simulink model "Voltage_Vector_with_script_fianl"  (R2024b)
settings: Solver=FixedStepAuto  StartTime=0.0  StopTime=0.5  FixedStep=1e-5  RelTol=1e-3
model workspace (MAT data in the model file):
  Cap = 0.004
  FL = 0.025
  Indcut = 0.005
  Initial_Voltage = 125
  R_Load = 1000
  V_dc = 300
  Vd = 125
  Vl = 400
  c = 125
  cap = 7.07e-05
  f_o = 50
  f_s = 5000
libraries: spsIGBTDiodeLib x72, spsSeriesRLCBranchLib x48, spsMultimeterLib x9, spsRMSLib x7, spsThreePhaseBreakerLib x6, spsTHDLib x6, spsThreePhaseSeriesRLCLoadLib x4, spsGroundLib x3, spsCurrentMeasurementLib x2, spsDCVoltageSourceLib x2, spsThreePhaseVIMeasurementLib x2, slpidlib x1
(part 3 of 3)

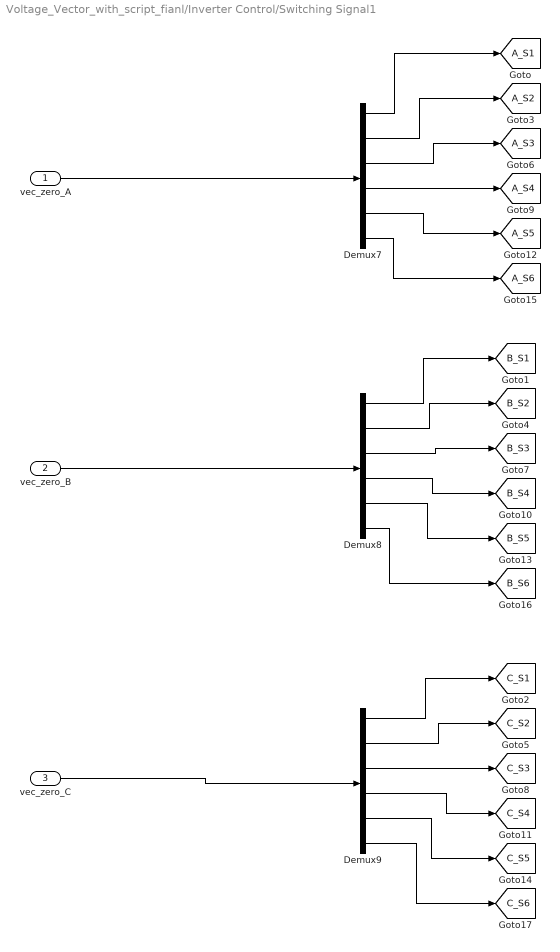
== system Voltage_Vector_with_script_fianl/Inverter Control/Switching Signal1 ==
  vec_zero_A : Inport
  vec_zero_B : Inport  Port=2
  vec_zero_C : Inport  Port=3
  Demux7 : Demux  Outputs=6
  Demux8 : Demux  Outputs=6
  Demux9 : Demux  Outputs=6
  tag scope: A_S1=global, A_S2=global, A_S3=global, A_S4=global, A_S5=global, A_S6=global, B_S1=global, B_S2=global, B_S3=global, B_S4=global, B_S5=global, B_S6=global, C_S1=global, C_S2=global, C_S3=global, C_S4=global, C_S5=global, C_S6=global
  wires:
  vec_zero_B/1 -> Demux8/1
  vec_zero_A/1 -> Demux7/1
  Demux8/2 -> [B_S2]
  Demux9/3 -> [C_S3]
  Demux8/4 -> [B_S4]
  vec_zero_C/1 -> Demux9/1
  Demux9/6 -> [C_S6]
  Demux7/2 -> [A_S2]
  Demux9/4 -> [C_S4]
  Demux7/4 -> [A_S4]
  Demux9/5 -> [C_S5]
  Demux9/1 -> [C_S1]
  Demux8/5 -> [B_S5]
  Demux7/3 -> [A_S3]
  Demux7/6 -> [A_S6]
  Demux9/2 -> [C_S2]
  Demux8/1 -> [B_S1]
  Demux8/3 -> [B_S3]
  Demux7/1 -> [A_S1]
  Demux8/6 -> [B_S6]
  Demux7/5 -> [A_S5]

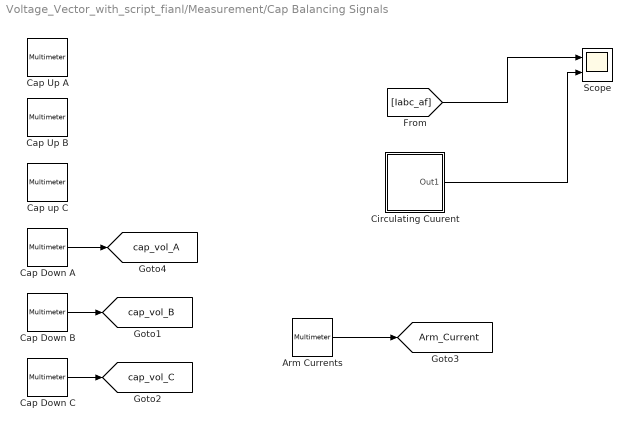
== system Voltage_Vector_with_script_fianl/Measurement/Cap Balancing Signals ==
  Arm Currents : spsMultimeterLib/Multimeter  L=86  sel=[46 48 50]  yselected={}  Gain=[1 1 1]  OutputType=Complex  PlotAtSimulationStop=on  PhasorSimulation=off
  Cap Down A : spsMultimeterLib/Multimeter  L=86  sel=[34 37 40 10 13 16]  yselected={}  Gain=[1 1 1 1 1 1]  OutputType=Complex  PlotAtSimulationStop=on  PhasorSimulation=off
  Cap Down B : spsMultimeterLib/Multimeter  L=86  sel=[35 38 41 11 14 17]  yselected={}  Gain=[1 1 1 1 1 1]  OutputType=Complex  PlotAtSimulationStop=on  PhasorSimulation=off
  Cap Down C : spsMultimeterLib/Multimeter  L=86  sel=[36 39 42 12 15 18]  yselected={}  Gain=[1 1 1 1 1 1]  OutputType=Complex  PlotAtSimulationStop=on  PhasorSimulation=off
  Cap Up A : spsMultimeterLib/Multimeter  L=86  sel=[7 19 22 25 28 31]  yselected={}  Gain=[1 1 1 1 1 1]  OutputType=Complex  PlotAtSimulationStop=off  PhasorSimulation=off
  Cap Up B : spsMultimeterLib/Multimeter  L=86  sel=[8 20 23 26 29 32]  yselected={}  Gain=[1 1 1 1 1 1]  OutputType=Complex  PlotAtSimulationStop=off  PhasorSimulation=off
  Cap up C : spsMultimeterLib/Multimeter  L=86  sel=[9 21 24 27 30 33]  yselected={}  Gain=[1 1 1 1 1 1]  OutputType=Complex  PlotAtSimulationStop=off  PhasorSimulation=off
  Circulating Cuurent : Subsystem
  Scope : Scope  NumInputPorts=2
  tag scope: Arm_Current=global, cap_vol_A=global, cap_vol_B=global, cap_vol_C=global
  wires:
  Cap Down A/1 -> [cap_vol_A]
  Cap Down B/1 -> [cap_vol_B]
  Cap Down C/1 -> [cap_vol_C]
  Arm Currents/1 -> [Arm_Current]
  [Iabc_af] -> Scope/1
  Circulating Cuurent/1(Out1) -> Scope/2

== system Voltage_Vector_with_script_fianl/Measurement/Current Measurements ==
  After Filtering : Subsystem
  Before Filtering : Subsystem

== system Voltage_Vector_with_script_fianl/Measurement/Voltage Measurements ==
  After Filtering : Subsystem
  Before Filtering : Subsystem
  Subsystem : Subsystem

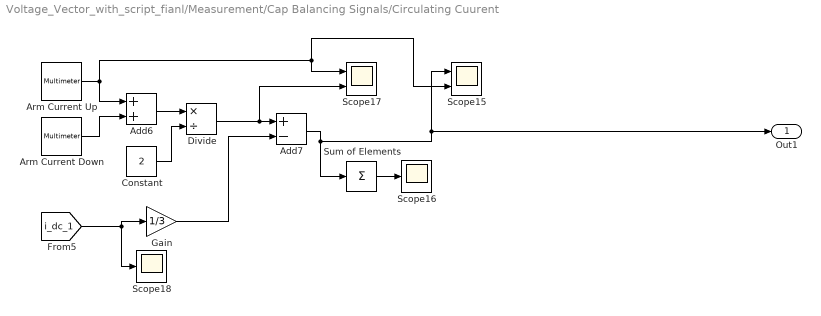
== system Voltage_Vector_with_script_fianl/Measurement/Cap Balancing Signals/Circulating Cuurent ==
  Add6 : Sum
  Add7 : Sum  Inputs=+-
  Arm Current Down : spsMultimeterLib/Multimeter  L=86  sel=[46 48 50]  yselected={}  Gain=[1 1 1]  OutputType=Complex  PlotAtSimulationStop=on  PhasorSimulation=off
  Arm Current Up : spsMultimeterLib/Multimeter  L=86  sel=[45 47 49]  yselected={}  Gain=[1 1 1]  OutputType=Complex  PlotAtSimulationStop=off  PhasorSimulation=off
  Constant : Constant  Value=2
  Divide : Product  Inputs=*/
  Gain : Gain  Gain=1/3
  Scope15 : Scope  NumInputPorts=2
  Scope16 : Scope
  Scope17 : Scope  NumInputPorts=2
  Scope18 : Scope
  Sum of Elements : Sum  Inputs=+
  Out1 : Outport
  wires:
  Gain/1 -> Add7/2
  Divide/1 -> Scope17/2, Add7/1
  Arm Current Up/1 -> Scope17/1, Scope15/2, Add6/1
  Add7/1 -> Sum of Elements/1, Out1/1, Scope15/1
  [i_dc_1] -> Gain/1, Scope18/1
  Add6/1 -> Divide/1
  Sum of Elements/1 -> Scope16/1
  Arm Current Down/1 -> Add6/2
  Constant/1 -> Divide/2

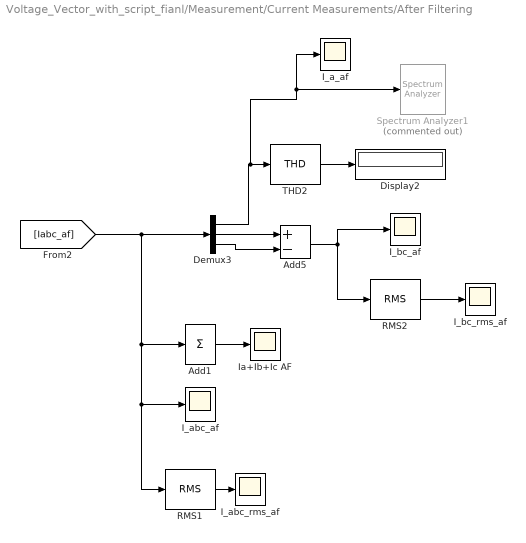
== system Voltage_Vector_with_script_fianl/Measurement/Current Measurements/After Filtering ==
  Add1 : Sum  Inputs=+
  Add5 : Sum  Inputs=+-
  Demux3 : Demux  Outputs=3
  Display2 : Display
  I_a_af : Scope
  I_abc_af : Scope
  I_abc_rms_af : Scope
  I_bc_af : Scope
  I_bc_rms_af : Scope
  Ia+Ib+Ic AF : Scope
  RMS1 : spsRMSLib/RMS  TrueRMS=on  Freq=50  RMSInit=120  Ts=0
  RMS2 : spsRMSLib/RMS  TrueRMS=on  Freq=50  RMSInit=120  Ts=0
  Spectrum Analyzer1 : SpectrumAnalyzer  Commented=on  WindowPosition=[1.000000,1.000000,1536.000000,840.000000,]  ScopeFrameLocation=window  ViewType=Spectrum and spectrogram  SampleRateSource=Property  SampleRate=44.1e3  PlotAsTwoSidedSpectrum=off  FrequencyScale=Log  RBW=50  FrequencySpan=Start and stop frequencies  StartFrequency=50  StopFrequency=20e3  YLimits=[-21.67839413,61.32124814]  ColorLimits=[-21.67839413,61.32124814]  SelectedToolstripTab=spectrumAnalyzerToolstrip.measurementsTab
  THD2 : spsTHDLib/THD  Freq=60  Ts=0
  wires:
  RMS1/1 -> I_abc_rms_af/1
  RMS2/1 -> I_bc_rms_af/1
  Demux3/2 -> Add5/1
  Add1/1 -> Ia+Ib+Ic AF/1
  Demux3/3 -> Add5/2
  THD2/1 -> Display2/1
  Demux3/1 -> THD2/1, Spectrum Analyzer1/1, I_a_af/1
  [Iabc_af] -> Demux3/1, Add1/1, I_abc_af/1, RMS1/1
  Add5/1 -> I_bc_af/1, RMS2/1

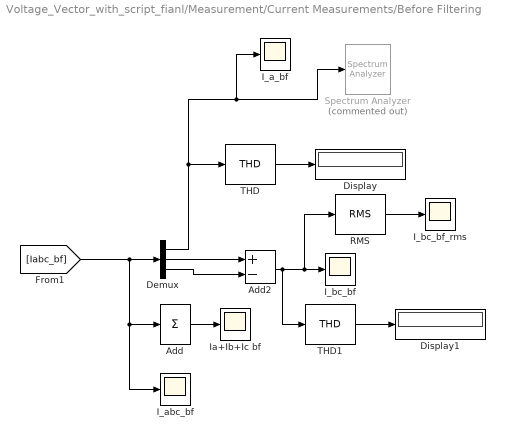
== system Voltage_Vector_with_script_fianl/Measurement/Current Measurements/Before Filtering ==
  Add : Sum  Inputs=+
  Add2 : Sum  Inputs=+-
  Demux : Demux  Outputs=3
  Display : Display
  Display1 : Display
  I_a_bf : Scope
  I_abc_bf : Scope
  I_bc_bf : Scope
  I_bc_bf_rms : Scope
  Ia+Ib+Ic bf : Scope
  RMS : spsRMSLib/RMS  TrueRMS=on  Freq=50  RMSInit=120  Ts=0
  Spectrum Analyzer : SpectrumAnalyzer  Commented=on  WindowPosition=[1.000000,1.000000,1536.000000,840.000000,]  ScopeFrameLocation=window  ViewType=Spectrum and spectrogram  SampleRateSource=Property  SampleRate=44.1e3  PlotAsTwoSidedSpectrum=off  FrequencyScale=Log  RBW=50  FrequencySpan=Start and stop frequencies  StartFrequency=50  StopFrequency=20e3  YLimits=[-37.25091553,62.23523651]  ColorLimits=[-37.25091553,62.23523651]  SelectedToolstripTab=spectrumAnalyzerToolstrip.measurementsTab
  THD : spsTHDLib/THD  Freq=60  Ts=0
  THD1 : spsTHDLib/THD  Freq=60  Ts=0
  wires:
  Add2/1 -> I_bc_bf/1, RMS/1, THD1/1
  THD1/1 -> Display1/1
  Demux/3 -> Add2/2
  Demux/2 -> Add2/1
  RMS/1 -> I_bc_bf_rms/1
  [Iabc_bf] -> Demux/1, Add/1, I_abc_bf/1
  Add/1 -> Ia+Ib+Ic bf/1
  Demux/1 -> THD/1, I_a_bf/1, Spectrum Analyzer/1
  THD/1 -> Display/1

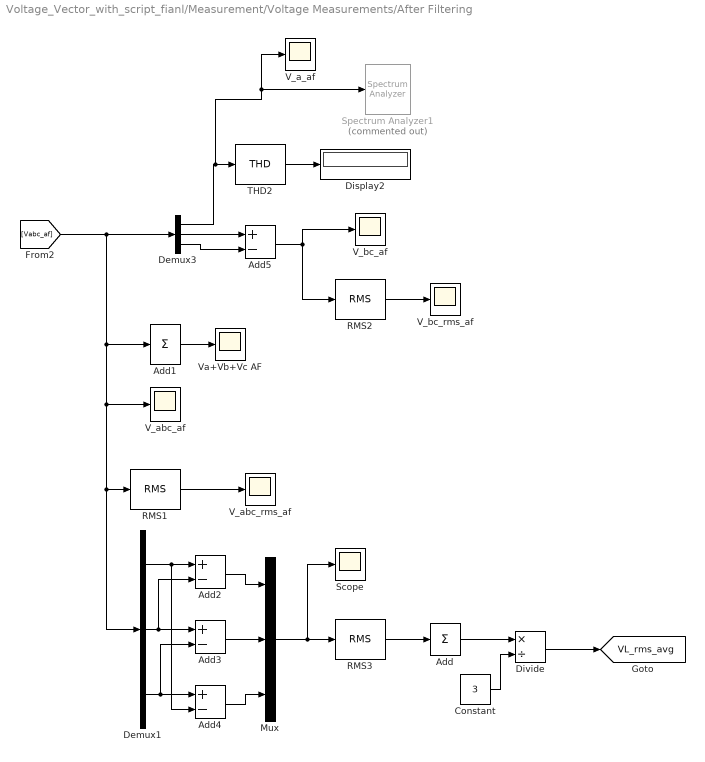
== system Voltage_Vector_with_script_fianl/Measurement/Voltage Measurements/After Filtering ==
  Add : Sum  Inputs=+
  Add1 : Sum  Inputs=+
  Add{2..5} (4 alike) : Sum  Inputs=+-
  Constant : Constant  Value=3
  Demux1 : Demux  Outputs=3
  Demux3 : Demux  Outputs=3
  Display2 : Display
  Divide : Product  Inputs=*/
  Mux : Mux  Inputs=3
  RMS1 : spsRMSLib/RMS  TrueRMS=on  Freq=50  RMSInit=120  Ts=0
  RMS2 : spsRMSLib/RMS  TrueRMS=on  Freq=50  RMSInit=120  Ts=0
  RMS3 : spsRMSLib/RMS  TrueRMS=on  Freq=50  RMSInit=0  Ts=0
  Scope : Scope
  Spectrum Analyzer1 : SpectrumAnalyzer  Commented=on  WindowPosition=[1.000000,1.000000,1536.000000,840.000000,]  ScopeFrameLocation=window  ViewType=Spectrum and spectrogram  SampleRateSource=Property  SampleRate=44.1e3  PlotAsTwoSidedSpectrum=off  FrequencyScale=Log  RBW=50  FrequencySpan=Start and stop frequencies  StartFrequency=50  StopFrequency=20e3  YLimits=[5.0325,80.7583]  ColorLimits=[5.0325,80.7583]  SelectedToolstripTab=spectrumAnalyzerToolstrip.measurementsTab
  THD2 : spsTHDLib/THD  Freq=50  Ts=0
  V_a_af : Scope
  V_abc_af : Scope
  V_abc_rms_af : Scope
  V_bc_af : Scope
  V_bc_rms_af : Scope
  Va+Vb+Vc AF : Scope
  tag scope: VL_rms_avg=global
  wires:
  Add5/1 -> RMS2/1, V_bc_af/1
  [Vabc_af] -> Demux1/1, RMS1/1, V_abc_af/1, Add1/1, Demux3/1
  Demux3/1 -> V_a_af/1, Spectrum Analyzer1/1, THD2/1
  THD2/1 -> Display2/1
  Demux3/3 -> Add5/2
  Add1/1 -> Va+Vb+Vc AF/1
  Demux3/2 -> Add5/1
  RMS2/1 -> V_bc_rms_af/1
  RMS1/1 -> V_abc_rms_af/1
  Add/1 -> Divide/1
  Constant/1 -> Divide/2
  Divide/1 -> [VL_rms_avg]
  Demux1/1 -> Add4/2, Add2/1
  Demux1/2 -> Add2/2, Add3/1
  Demux1/3 -> Add3/2, Add4/1
  Add3/1 -> Mux/2
  Add2/1 -> Mux/1
  Add4/1 -> Mux/3
  Mux/1 -> Scope/1, RMS3/1
  RMS3/1 -> Add/1

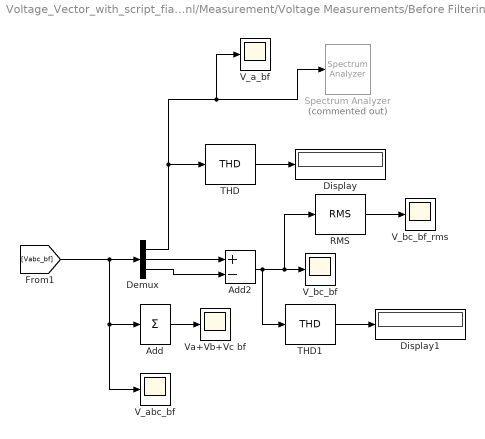
== system Voltage_Vector_with_script_fianl/Measurement/Voltage Measurements/Before Filtering ==
  Add : Sum  Inputs=+
  Add2 : Sum  Inputs=+-
  Demux : Demux  Outputs=3
  Display : Display
  Display1 : Display
  RMS : spsRMSLib/RMS  TrueRMS=on  Freq=50  RMSInit=120  Ts=0
  Spectrum Analyzer : SpectrumAnalyzer  Commented=on  WindowPosition=[1.000000,1.000000,1536.000000,840.000000,]  ScopeFrameLocation=window  ViewType=Spectrum and spectrogram  SampleRateSource=Property  SampleRate=44.1e3  PlotAsTwoSidedSpectrum=off  FrequencyScale=Log  RBW=50  FrequencySpan=Start and stop frequencies  StartFrequency=50  StopFrequency=20e3  YLimits=[-20.56239862,87.43260692]  ColorLimits=[-20.56239862,87.43260692]  SelectedToolstripTab=spectrumAnalyzerToolstrip.measurementsTab
  THD : spsTHDLib/THD  Freq=50  Ts=0
  THD1 : spsTHDLib/THD  Freq=50  Ts=0
  V_a_bf : Scope
  V_abc_bf : Scope
  V_bc_bf : Scope
  V_bc_bf_rms : Scope
  Va+Vb+Vc bf : Scope
  wires:
  THD/1 -> Display/1
  Demux/1 -> Spectrum Analyzer/1, V_a_bf/1, THD/1
  Add/1 -> Va+Vb+Vc bf/1
  [Vabc_bf] -> V_abc_bf/1, Add/1, Demux/1
  RMS/1 -> V_bc_bf_rms/1
  Demux/2 -> Add2/1
  Demux/3 -> Add2/2
  THD1/1 -> Display1/1
  Add2/1 -> THD1/1, RMS/1, V_bc_bf/1

== system Voltage_Vector_with_script_fianl/Measurement/Voltage Measurements/Subsystem ==
  Add : Sum  Inputs=+-
  Add1 : Sum  Inputs=+-
  Demux : Demux  Outputs=3
  Demux1 : Demux  Outputs=3
  Scope : Scope  NumInputPorts=3
  Scope1 : Scope  NumInputPorts=3
  wires:
  [Vabc_af] -> Scope1/1, Demux1/1
  [Vabc_bf] -> Demux/1, Scope/1
  Demux/1 -> Scope/2
  Demux1/1 -> Scope1/2
  Add/1 -> Scope/3
  Add1/1 -> Scope1/3
  Demux/2 -> Add/1
  Demux/3 -> Add/2
  Demux1/2 -> Add1/1
  Demux1/3 -> Add1/2

== matlab function Voltage_Vector_with_script_fianl/Inverter Control/MATLAB Function3 ==
  data: tita_k output; tita input; CV_1 output; CV_2 output; CV_3 output; T output; V_L input; Vd_ input; f input; fs input
function [tita_k, CV_1, CV_2, CV_3, T] = fnc(tita,V_L,Vd_,f,fs)

Ts = 1/fs;

% Transform matrix
A = [1 0 0.5; cos(2*pi/3) sin(2*pi/3) 0.5; cos(4*pi/3) sin(4*pi/3) 0.5]; % Transform matrix
B = [cos(0) cos(2*pi/3) cos(4*pi/3); sin(0) sin(2*pi/3) sin(4*pi/3)];

% Model Parameter
% corner_vec = zeros(1,10);
% dwell_time = zeros(1,4);

% Calculations

r_k = sqrt(6)*V_L / 2;

% tita_k = floor(tita*fs/(f*360))*360*f/fs;
tita_k = tita - mod(tita, 360*f/fs);

x = [r_k*cos(deg2rad(tita_k)); r_k*sin(deg2rad(tita_k)); 0];
V_pole = (2/3)*A*x;
Vnor = V_pole' / Vd_;
% corner_vec(1,1) = tita_k;
% dwell_time(1,1) = tita_k;

% conor vector calculation

CV = Vnor +3;
CV_1 = floor(CV);
error = CV - floor(CV);
[~,i_1] = max(error); % ~ represent the magnitude but ~ neglecte it; i is the index(position), In for loop we can find the magnitude and index
CV_2 = CV_1;
CV_2(i_1) = CV_2(i_1) + 1;
error(i_1) = 0;

[~,i_2] = max(error); % i think max function is not nessaccery , we can you only error
CV_3 = CV_2;
CV_3(i_2) = CV_3(i_2) + 1;
CV_M = [CV_1' CV_2' CV_3'];

temp = [Vd_*B*CV_M; 1 1 1];% first find the Vd*B*CV_M matrix and then add the 1 1 1 row to it.
Y = Ts*[r_k*cos(deg2rad(tita_k));r_k*sin(deg2rad(tita_k)); 1];
T = abs(temp\Y);
           
% corner_vec(1,2:end) = reshape(CV_M, 1, []);
% dwell_time(1,2:end) = T;

== matlab function Voltage_Vector_with_script_fianl/Inverter Control/MATLAB Function2 ==
  data: t input; tita output; fo input; ini_tita input
function tita = fcn(t, fo, ini_tita)

angle = t * fo * 360 + ini_tita;
tita = mod(angle,360);

== matlab function Voltage_Vector_with_script_fianl/Inverter Control/MATLAB Function ==
  data: CV input; vec_zero_A output; cap_vol_a input; cap_vol_b input; cap_vol_c input; arm_cu input; vec_zero_B output; vec_zero_C output
function [vec_zero_A,vec_zero_B,vec_zero_C] = sec_cap(CV, cap_vol_a, cap_vol_b, cap_vol_c, arm_cu)

low_cap_ind_A = 0;
low_cap_ind_B = 0;
low_cap_ind_C = 0;

[~, original_indexes_a] = sort(cap_vol_a); % capacitor voltages tika sort karanawa.
[~, original_indexes_b]  = sort(cap_vol_b);
[~, original_indexes_c]  = sort(cap_vol_c);

cv_a = CV(1); % lower arm eke on wenna ona capacitors ganana.
cv_b = CV(2);
cv_c = CV(3);

arm_cu_A = arm_cu(1); % arm current tika wen karagannawa.
arm_cu_B = arm_cu(2);
arm_cu_C = arm_cu(3);

low_n_A = cv_a; % upper arm eken operate wenna ona capacitors ganana.
low_n_B = cv_b;
low_n_C = cv_c;

vec_zero_A = zeros(1,6)';
vec_zero_B = zeros(1,6)';
vec_zero_C = zeros(1,6)';

% if Time_ps == 0

%----------------------------------------------------------------
if arm_cu_A > 0

    % select the capacitors that voltages are minimum
    low_cap_ind_A = original_indexes_a(1:low_n_A);
    var = low_cap_ind_A;
    for i = 1 : low_n_A
        % up_cap_ind_A = var(i);
        vec_zero_A(var(i)) = 1;
    end

else
    % select the capacitors that voltages are maximum
    low_cap_ind_A = flip(original_indexes_a);
    low_cap_ind_A = low_cap_ind_A(1:low_n_A);
    var = low_cap_ind_A;
    for i = 1 : low_n_A
        % up_cap_ind_A = var(i);
        vec_zero_A(var(i)) = 1;
    end
end

%-----------------------------------------------------------------

if arm_cu_B > 0

    % select the capacitors that voltages are minimum
    low_cap_ind_B = original_indexes_b(1:low_n_B);
    var = low_cap_ind_B;
    for i = 1 : low_n_B
        % up_cap_ind_B = var(i);
        vec_zero_B(var(i)) = 1;
    end        

else
    % select the capacitors that voltages are maximum
    low_cap_ind_B = flip(original_indexes_b);
    low_cap_ind_B = low_cap_ind_B(1:low_n_B);
    var = low_cap_ind_B;
    for i = 1 : low_n_B
        % up_cap_ind_B = var(i);
        vec_zero_B(var(i)) = 1;
    end        
end

%----------------------------------------------------------------
if arm_cu_C > 0

    % select the capacitors that voltages are minimum
    low_cap_ind_C = original_indexes_c(1:low_n_C);
    var = low_cap_ind_C;
    for i = 1 : low_n_C
        % up_cap_ind_C = var(i);
        vec_zero_C(var(i)) = 1;
    end

else
    % select the capacitors that voltages are maximum
    low_cap_ind_C = flip(original_indexes_c);
    low_cap_ind_C = low_cap_ind_C(1:low_n_C);
    var = low_cap_ind_C;
    for i = 1 : low_n_C
        % up_cap_ind_C = var(i);
        vec_zero_C(var(i)) = 1;
    end
end
%----------------------------------------------------------------

end


% end

== matlab function Voltage_Vector_with_script_fianl/Inverter Control/Sorting Algorith1 ==
  data: t input; CV_1 input; CV_2 input; CV_3 input; T input; fs input; CV output; time_PS output
function [CV ,time_PS] = FN1(t,CV_1,CV_2,CV_3,T,fs)
    time_PS = mod(t,1/fs); % Time per sample
   
    if time_PS<= T(1) / 2
        % from t=0 to t=T(1) the first corner vector must be presented
        CV = CV_1;
        
    elseif time_PS <= T(1) / 2 + T(2) / 2
        % from t=T(1) to t=T(2) the second corner vector must be presented
        CV = CV_2;

    elseif time_PS <= T(1) / 2 + T(2) / 2 + T(3)
        % from t=T(1) to t=T(2) the second corner vector must be presented
        CV = CV_3;
        
    elseif time_PS <= T(1) / 2 + T(2) + T(3)
        % from t=T(1) to t=T(2) the second corner vector must be presented
        CV = CV_2;
    else
        % from t=T(2) to t=T(3) the third corner vector must be presented
        CV = CV_1;
    end
end

== matlab function Voltage_Vector_with_script_fianl/Inverter Control/MATLAB Function1 ==
  data: Arm_current input; A_C1 output; A_C2 output; A_C3 output
function [A_C1,A_C2,A_C3] = fcn(Arm_current)

A_C1 = Arm_current(1);
A_C2 = Arm_current(2);
A_C3 = Arm_current(3);

end
